simulink model "Seat_Belt1"  (R2025b)
settings: Solver=VariableStepAuto  StartTime=0.0  StopTime=inf  RelTol=1e-3
settings Model: Creator=Pai  LastModifiedBy=Pai

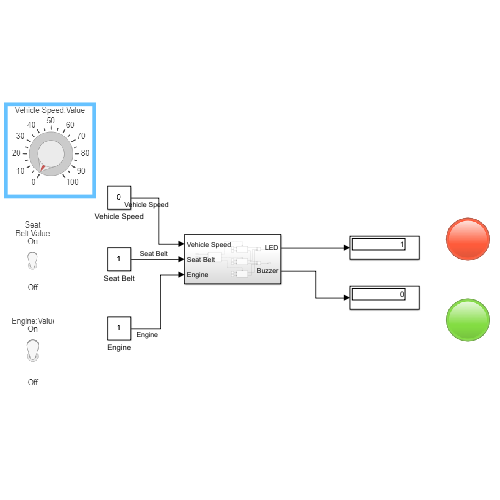
[thumbnail: Simulink's stored preview of the top-level diagram]
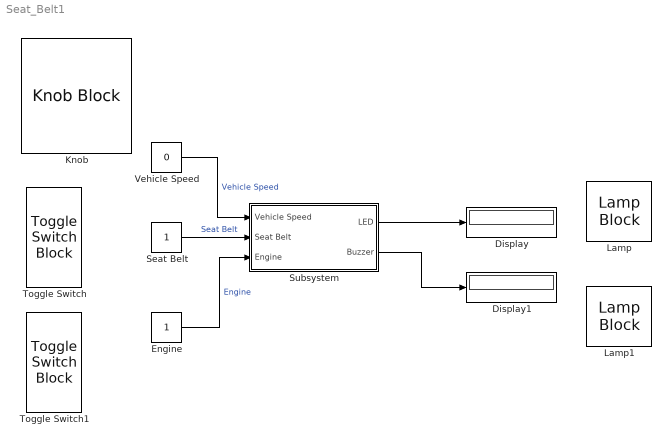
== system Seat_Belt1 ==
  Display : Display
  Display1 : Display
  Engine : Constant
  Knob : KnobBlock
  Lamp : LampBlock  LabelPosition=Hide  DefaultColor=[192.0, 192.0, 192.0]
  Lamp1 : LampBlock  LabelPosition=Hide  DefaultColor=[192.0, 192.0, 192.0]
  Seat Belt : Constant
  Subsystem : Subsystem
  Toggle Switch : ToggleSwitchBlock
  Toggle Switch1 : ToggleSwitchBlock
  Vehicle Speed : Constant  Value=0
  wires:
  Vehicle Speed/1 -> Subsystem/1(Vehicle Speed)  "Vehicle Speed"
  Subsystem/1(LED) -> Display/1
  Seat Belt/1 -> Subsystem/2(Seat Belt)  "Seat Belt"
  Subsystem/2(Buzzer) -> Display1/1
  Engine/1 -> Subsystem/3(Engine)  "Engine"

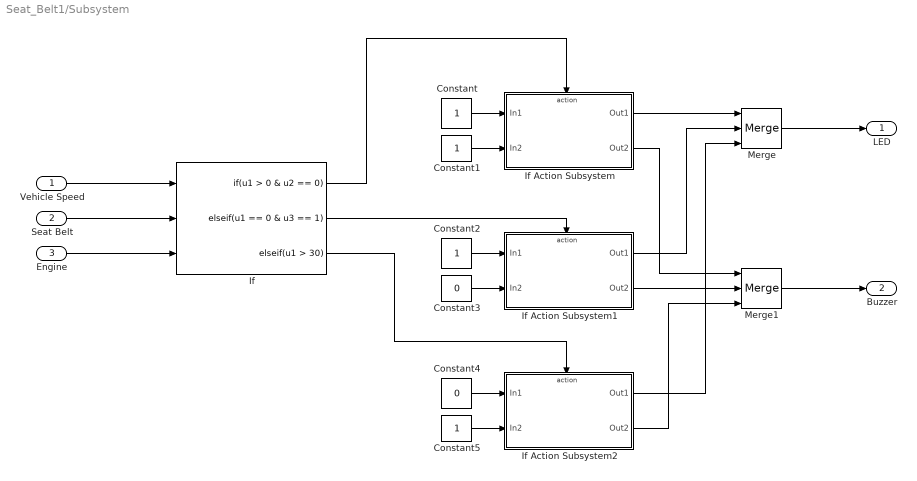
== system Seat_Belt1/Subsystem ==
  Vehicle Speed : Inport
  Seat Belt : Inport  Port=2
  Engine : Inport  Port=3
  Constant{,1..2,5} (4 alike) : Constant
  Constant3 : Constant  Value=0
  Constant4 : Constant  Value=0
  If : If  NumInputs=3  IfExpression=u1 > 0 & u2 == 0  ElseIfExpressions=u1 == 0 & u3 == 1,u1 > 30  ShowElse=off
  If Action Subsystem : Subsystem  TreatAsAtomicUnit=on
  If Action Subsystem1 : Subsystem  TreatAsAtomicUnit=on
  If Action Subsystem2 : Subsystem  TreatAsAtomicUnit=on
  Merge : Merge  Inputs=3
  Merge1 : Merge  Inputs=3
  LED : Outport
  Buzzer : Outport  Port=2
  wires:
  Vehicle Speed/1 -> If/1
  Seat Belt/1 -> If/2
  Engine/1 -> If/3
  If/1 -> If Action Subsystem/Action
  Constant/1 -> If Action Subsystem/1(In1)
  Constant1/1 -> If Action Subsystem/2(In2)
  Constant2/1 -> If Action Subsystem1/1(In1)
  If/2 -> If Action Subsystem1/Action
  Constant3/1 -> If Action Subsystem1/2(In2)
  Constant4/1 -> If Action Subsystem2/1(In1)
  If/3 -> If Action Subsystem2/Action
  Constant5/1 -> If Action Subsystem2/2(In2)
  If Action Subsystem/1(Out1) -> Merge/1
  If Action Subsystem1/1(Out1) -> Merge/2
  If Action Subsystem2/1(Out1) -> Merge/3
  If Action Subsystem/2(Out2) -> Merge1/1
  If Action Subsystem1/2(Out2) -> Merge1/2
  If Action Subsystem2/2(Out2) -> Merge1/3
  Merge/1 -> LED/1
  Merge1/1 -> Buzzer/1

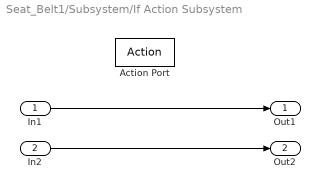
== system Seat_Belt1/Subsystem/If Action Subsystem ==
  In1 : Inport
  In2 : Inport  Port=2
  Action Port : ActionPort  ActionPortLabel=if(u1 > 0 & u2 == 0)
  Out1 : Outport
  Out2 : Outport  Port=2
  wires:
  In1/1 -> Out1/1
  In2/1 -> Out2/1

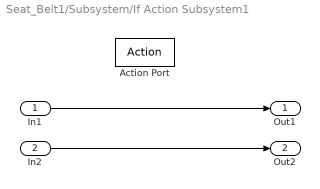
== system Seat_Belt1/Subsystem/If Action Subsystem1 ==
  In1 : Inport
  In2 : Inport  Port=2
  Action Port : ActionPort  ActionPortLabel=elseif(u1 == 0 & u3 == 1)
  Out1 : Outport
  Out2 : Outport  Port=2
  wires:
  In1/1 -> Out1/1
  In2/1 -> Out2/1

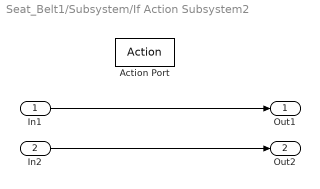
== system Seat_Belt1/Subsystem/If Action Subsystem2 ==
  In1 : Inport
  In2 : Inport  Port=2
  Action Port : ActionPort  ActionPortLabel=elseif(u1 > 30)
  Out1 : Outport
  Out2 : Outport  Port=2
  wires:
  In1/1 -> Out1/1
  In2/1 -> Out2/1
